simulink model "Inverter_Trifase_PWM_23"  (R2023b)
settings: Solver=ode23s  StartTime=0.0  StopTime=5
values from neighbouring files (symbols this model uses):
  Lc = 10e-3    (= 0.01)    [data.m]
  Rc = 20    [data.m]
  tau = 0.1    [data.m]
  Tc = 100e-6    (= 0.0001)    [data.m]
undefined symbols (not defined in the file or in its folder): DiscIntNeverNeededParam
libraries: fl_lib x80, nesl_utility x51, slpidlib x3, simulink x1
(part 2 of 2)

== system Inverter_Trifase_PWM_23/load ==
  Capacitor : fl_lib/Electrical/Electrical Elements/Capacitor  c=Cc F  r=1e-6 Ohm  g=0 1/Ohm  i_specify=off  i_priority=None  i=0 A  i_nominal_specify=off  i_nominal_value=1  i_nominal_unit=A  v_specify=off  v_priority=None  v=0 V  v_nominal_specify=off  v_nominal_value=1  v_nominal_unit=V  vc_specify=off  vc_priority=High  vc=0 V  vc_nominal_specify=off  vc_nominal_value=1  vc_nominal_unit=V
  Capacitor1 : fl_lib/Electrical/Electrical Elements/Capacitor  c=Cc F  r=1e-6 Ohm  g=0 1/Ohm  i_specify=off  i_priority=None  i=0 A  i_nominal_specify=off  i_nominal_value=1  i_nominal_unit=A  v_specify=off  v_priority=None  v=0 V  v_nominal_specify=off  v_nominal_value=1  v_nominal_unit=V  vc_specify=off  vc_priority=High  vc=0 V  vc_nominal_specify=off  vc_nominal_value=1  vc_nominal_unit=V
  Capacitor2 : fl_lib/Electrical/Electrical Elements/Capacitor  c=Cc F  r=1e-6 Ohm  g=0 1/Ohm  i_specify=off  i_priority=None  i=0 A  i_nominal_specify=off  i_nominal_value=1  i_nominal_unit=A  v_specify=off  v_priority=None  v=0 V  v_nominal_specify=off  v_nominal_value=1  v_nominal_unit=V  vc_specify=off  vc_priority=High  vc=0 V  vc_nominal_specify=off  vc_nominal_value=1  vc_nominal_unit=V
  Electrical Reference1 : fl_lib/Electrical/Electrical Elements/Electrical Reference
  Inductor : fl_lib/Electrical/Electrical Elements/Inductor  l=Lc H  r=0 Ohm  g=1e-9 1/Ohm  i_specify=off  i_priority=None  i=0 A  i_nominal_specify=off  i_nominal_value=1  i_nominal_unit=A  v_specify=off  v_priority=None  v=0 V  v_nominal_specify=off  v_nominal_value=1  v_nominal_unit=V  i_L_specify=on  i_L_priority=High  i_L=0 A  i_L_nominal_specify=off  i_L_nominal_value=1  i_L_nominal_unit=A
  Inductor1 : fl_lib/Electrical/Electrical Elements/Inductor  l=Lc H  r=0 Ohm  g=1e-9 1/Ohm  i_specify=off  i_priority=None  i=0 A  i_nominal_specify=off  i_nominal_value=1  i_nominal_unit=A  v_specify=off  v_priority=None  v=0 V  v_nominal_specify=off  v_nominal_value=1  v_nominal_unit=V  i_L_specify=on  i_L_priority=High  i_L=0 A  i_L_nominal_specify=off  i_L_nominal_value=1  i_L_nominal_unit=A
  Inductor2 : fl_lib/Electrical/Electrical Elements/Inductor  l=Lc H  r=0 Ohm  g=1e-9 1/Ohm  i_specify=off  i_priority=None  i=0 A  i_nominal_specify=off  i_nominal_value=1  i_nominal_unit=A  v_specify=off  v_priority=None  v=0 V  v_nominal_specify=off  v_nominal_value=1  v_nominal_unit=V  i_L_specify=on  i_L_priority=High  i_L=0 A  i_L_nominal_specify=off  i_L_nominal_value=1  i_L_nominal_unit=A
  Resistor : fl_lib/Electrical/Electrical Elements/Resistor  R=Rc Ohm  i_specify=off  i_priority=None  i=0 A  i_nominal_specify=off  i_nominal_value=1  i_nominal_unit=A  v_specify=off  v_priority=None  v=0 V  v_nominal_specify=off  v_nominal_value=1  v_nominal_unit=V
  Resistor1 : fl_lib/Electrical/Electrical Elements/Resistor  R=Rc Ohm  i_specify=off  i_priority=None  i=0 A  i_nominal_specify=off  i_nominal_value=1  i_nominal_unit=A  v_specify=off  v_priority=None  v=0 V  v_nominal_specify=off  v_nominal_value=1  v_nominal_unit=V
  Resistor2 : fl_lib/Electrical/Electrical Elements/Resistor  R=Rc Ohm  i_specify=off  i_priority=None  i=0 A  i_nominal_specify=off  i_nominal_value=1  i_nominal_unit=A  v_specify=off  v_priority=None  v=0 V  v_nominal_specify=off  v_nominal_value=1  v_nominal_unit=V
  A : PMIOPort  Side=Left
  B : PMIOPort  Port=2  Side=Left
  C : PMIOPort  Port=3  Side=Left
  connections:
  Inductor/RConn1 -- Electrical Reference1/LConn1 -- Inductor2/RConn1 -- Inductor1/RConn1
  Inductor/LConn1 -- Resistor/RConn1
  Inductor1/LConn1 -- Resistor1/RConn1
  Inductor2/LConn1 -- Resistor2/RConn1
  Capacitor/LConn1 -- A/RConn1
  Capacitor/RConn1 -- Resistor/LConn1
  Capacitor1/LConn1 -- B/RConn1
  Capacitor1/RConn1 -- Resistor1/LConn1
  Capacitor2/LConn1 -- C/RConn1
  Capacitor2/RConn1 -- Resistor2/LConn1

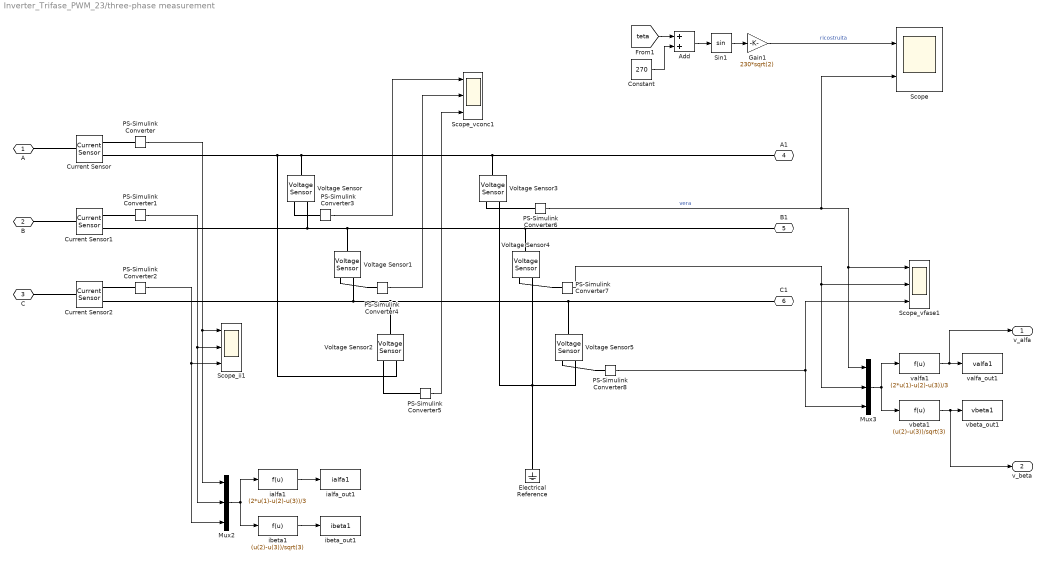
== system Inverter_Trifase_PWM_23/three-phase measurement ==
  Add : Sum
  Constant : Constant  Value=270
  Current Sensor : fl_lib/Electrical/Electrical Sensors/Current Sensor
  Current Sensor1 : fl_lib/Electrical/Electrical Sensors/Current Sensor
  Current Sensor2 : fl_lib/Electrical/Electrical Sensors/Current Sensor
  Electrical Reference : fl_lib/Electrical/Electrical Elements/Electrical Reference
  Gain1 : Gain  Gain=230*sqrt(2)
  Mux2 : Mux  Inputs=3
  Mux3 : Mux  Inputs=3
  PS-Simulink Converter{,1..8} (9 alike) : nesl_utility/PS-Simulink Converter  PhysicalDomain=network_engine_domain  SubClassName=ps_output  LeftPortType=input  RightPortType=output  PseudoPeriodic=off  Frequencies=[]  VectorFormat=inherit  Unit=inherit  AffineConversion=off
  Scope : Scope  NumInputPorts=2
  Scope_ii1 : Scope  NumInputPorts=3
  Scope_vconc1 : Scope  NumInputPorts=3
  Scope_vfase1 : Scope  NumInputPorts=3
  Sin1 : Trigonometry
  Voltage Sensor{,1..5} (6 alike) : fl_lib/Electrical/Electrical Sensors/Voltage Sensor
  ialfa1 : Fcn  Expr=(2*u(1)-u(2)-u(3))/3
  ialfa_out1 : ToWorkspace  VariableName=ialfa1  SampleTime=-1
  ibeta1 : Fcn  Expr=(u(2)-u(3))/sqrt(3)
  ibeta_out1 : ToWorkspace  VariableName=ibeta1  SampleTime=-1
  valfa1 : Fcn  Expr=(2*u(1)-u(2)-u(3))/3
  valfa_out1 : ToWorkspace  VariableName=valfa1  SampleTime=-1
  vbeta1 : Fcn  Expr=(u(2)-u(3))/sqrt(3)
  vbeta_out1 : ToWorkspace  VariableName=vbeta1  SampleTime=-1
  A : PMIOPort  Side=Left
  B : PMIOPort  Port=2  Side=Left
  C : PMIOPort  Port=3  Side=Left
  A1 : PMIOPort  Port=4  Side=Right
  B1 : PMIOPort  Port=5  Side=Right
  C1 : PMIOPort  Port=6  Side=Right
  v_alfa : Outport
  v_beta : Outport  Port=2
  wires:
  ibeta1/1 -> ibeta_out1/1
  ialfa1/1 -> ialfa_out1/1
  Mux2/1 -> ialfa1/1, ibeta1/1
  PS-Simulink Converter2/1 -> Scope_ii1/3, Mux2/3
  PS-Simulink Converter1/1 -> Scope_ii1/2, Mux2/2
  PS-Simulink Converter/1 -> Scope_ii1/1, Mux2/1
  PS-Simulink Converter3/1 -> Scope_vconc1/1
  PS-Simulink Converter4/1 -> Scope_vconc1/2
  PS-Simulink Converter5/1 -> Scope_vconc1/3
  vbeta1/1 -> v_beta/1, vbeta_out1/1
  valfa1/1 -> v_alfa/1, valfa_out1/1
  Mux3/1 -> valfa1/1, vbeta1/1
  PS-Simulink Converter6/1 -> Scope/2, Scope_vfase1/1, Mux3/1  "vera"
  PS-Simulink Converter7/1 -> Scope_vfase1/2, Mux3/2
  PS-Simulink Converter8/1 -> Mux3/3, Scope_vfase1/3
  Gain1/1 -> Scope/1  "ricostruita"
  Sin1/1 -> Gain1/1
  Constant/1 -> Add/2
  [teta] -> Add/1
  Add/1 -> Sin1/1
  connections:
  Current Sensor/LConn1 -- A/RConn1
  Current Sensor1/LConn1 -- B/RConn1
  C/RConn1 -- Current Sensor2/LConn1
  PS-Simulink Converter/LConn1 -- Current Sensor/RConn1
  PS-Simulink Converter1/LConn1 -- Current Sensor1/RConn1
  PS-Simulink Converter2/LConn1 -- Current Sensor2/RConn1
  A1/RConn1 -- Voltage Sensor3/LConn1 -- Voltage Sensor/LConn1 -- Voltage Sensor2/RConn2 -- Current Sensor/RConn2
  B1/RConn1 -- Voltage Sensor1/LConn1 -- Voltage Sensor/RConn2 -- Current Sensor1/RConn2 -- Voltage Sensor4/LConn1
  C1/RConn1 -- Voltage Sensor5/LConn1 -- Voltage Sensor2/LConn1 -- Voltage Sensor1/RConn2 -- Current Sensor2/RConn2
  PS-Simulink Converter3/LConn1 -- Voltage Sensor/RConn1
  PS-Simulink Converter4/LConn1 -- Voltage Sensor1/RConn1
  PS-Simulink Converter5/LConn1 -- Voltage Sensor2/RConn1
  Voltage Sensor3/RConn2 -- Electrical Reference/LConn1 -- Voltage Sensor5/RConn2 -- Voltage Sensor4/RConn2
  PS-Simulink Converter6/LConn1 -- Voltage Sensor3/RConn1
  PS-Simulink Converter7/LConn1 -- Voltage Sensor4/RConn1
  PS-Simulink Converter8/LConn1 -- Voltage Sensor5/RConn1

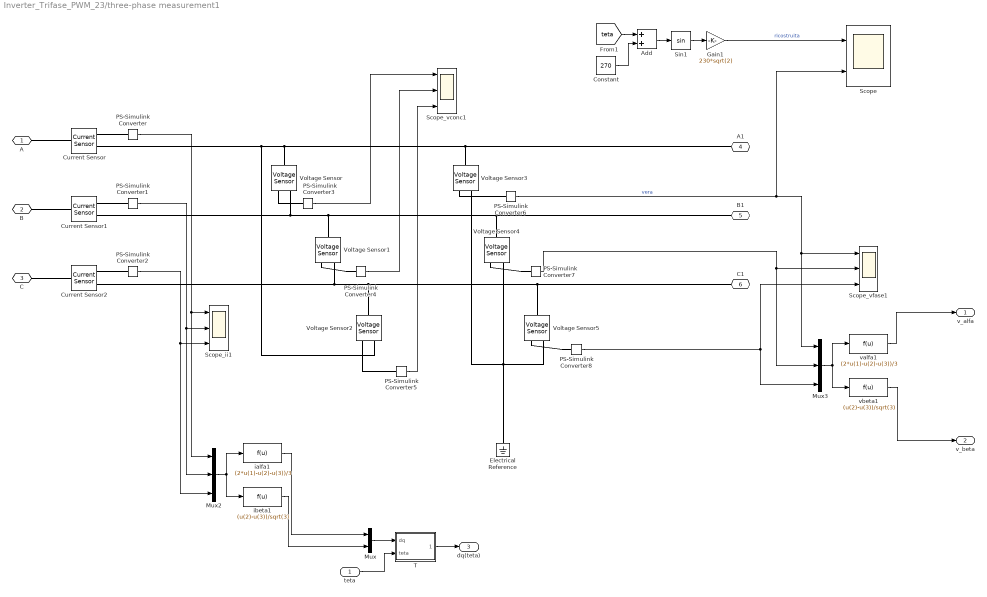
== system Inverter_Trifase_PWM_23/three-phase measurement1 ==
  teta : Inport
  Add : Sum
  Constant : Constant  Value=270
  Current Sensor : fl_lib/Electrical/Electrical Sensors/Current Sensor
  Current Sensor1 : fl_lib/Electrical/Electrical Sensors/Current Sensor
  Current Sensor2 : fl_lib/Electrical/Electrical Sensors/Current Sensor
  Electrical Reference : fl_lib/Electrical/Electrical Elements/Electrical Reference
  Gain1 : Gain  Gain=230*sqrt(2)
  Mux : Mux  Inputs=2
  Mux2 : Mux  Inputs=3
  Mux3 : Mux  Inputs=3
  PS-Simulink Converter{,1..8} (9 alike) : nesl_utility/PS-Simulink Converter  PhysicalDomain=network_engine_domain  SubClassName=ps_output  LeftPortType=input  RightPortType=output  PseudoPeriodic=off  Frequencies=[]  VectorFormat=inherit  Unit=inherit  AffineConversion=off
  Scope : Scope  NumInputPorts=2
  Scope_ii1 : Scope  NumInputPorts=3
  Scope_vconc1 : Scope  NumInputPorts=3
  Scope_vfase1 : Scope  NumInputPorts=3
  Sin1 : Trigonometry
  T : Subsystem
  Voltage Sensor{,1..5} (6 alike) : fl_lib/Electrical/Electrical Sensors/Voltage Sensor
  ialfa1 : Fcn  Expr=(2*u(1)-u(2)-u(3))/3
  ibeta1 : Fcn  Expr=(u(2)-u(3))/sqrt(3)
  valfa1 : Fcn  Expr=(2*u(1)-u(2)-u(3))/3
  vbeta1 : Fcn  Expr=(u(2)-u(3))/sqrt(3)
  A : PMIOPort  Side=Left
  B : PMIOPort  Port=2  Side=Left
  C : PMIOPort  Port=3  Side=Left
  A1 : PMIOPort  Port=4  Side=Right
  B1 : PMIOPort  Port=5  Side=Right
  C1 : PMIOPort  Port=6  Side=Right
  v_alfa : Outport
  v_beta : Outport  Port=2
  dq(teta) : Outport  Port=3
  wires:
  ibeta1/1 -> Mux/2
  ialfa1/1 -> Mux/1
  Mux2/1 -> ialfa1/1, ibeta1/1
  PS-Simulink Converter2/1 -> Scope_ii1/3, Mux2/3
  PS-Simulink Converter1/1 -> Scope_ii1/2, Mux2/2
  PS-Simulink Converter/1 -> Scope_ii1/1, Mux2/1
  PS-Simulink Converter3/1 -> Scope_vconc1/1
  PS-Simulink Converter4/1 -> Scope_vconc1/2
  PS-Simulink Converter5/1 -> Scope_vconc1/3
  vbeta1/1 -> v_beta/1
  valfa1/1 -> v_alfa/1
  Mux3/1 -> valfa1/1, vbeta1/1
  PS-Simulink Converter6/1 -> Scope/2, Scope_vfase1/1, Mux3/1  "vera"
  PS-Simulink Converter7/1 -> Scope_vfase1/2, Mux3/2
  PS-Simulink Converter8/1 -> Mux3/3, Scope_vfase1/3
  Gain1/1 -> Scope/1  "ricostruita"
  Sin1/1 -> Gain1/1
  Constant/1 -> Add/2
  [teta] -> Add/1
  Add/1 -> Sin1/1
  Mux/1 -> T/1(dq)
  teta/1 -> T/2(teta)
  T/1(dq(teta)) -> dq(teta)/1
  connections:
  Current Sensor/LConn1 -- A/RConn1
  Current Sensor1/LConn1 -- B/RConn1
  C/RConn1 -- Current Sensor2/LConn1
  PS-Simulink Converter/LConn1 -- Current Sensor/RConn1
  PS-Simulink Converter1/LConn1 -- Current Sensor1/RConn1
  PS-Simulink Converter2/LConn1 -- Current Sensor2/RConn1
  A1/RConn1 -- Voltage Sensor3/LConn1 -- Voltage Sensor/LConn1 -- Voltage Sensor2/RConn2 -- Current Sensor/RConn2
  B1/RConn1 -- Voltage Sensor1/LConn1 -- Voltage Sensor/RConn2 -- Current Sensor1/RConn2 -- Voltage Sensor4/LConn1
  C1/RConn1 -- Voltage Sensor5/LConn1 -- Voltage Sensor2/LConn1 -- Voltage Sensor1/RConn2 -- Current Sensor2/RConn2
  PS-Simulink Converter3/LConn1 -- Voltage Sensor/RConn1
  PS-Simulink Converter4/LConn1 -- Voltage Sensor1/RConn1
  PS-Simulink Converter5/LConn1 -- Voltage Sensor2/RConn1
  Voltage Sensor3/RConn2 -- Electrical Reference/LConn1 -- Voltage Sensor5/RConn2 -- Voltage Sensor4/RConn2
  PS-Simulink Converter6/LConn1 -- Voltage Sensor3/RConn1
  PS-Simulink Converter7/LConn1 -- Voltage Sensor4/RConn1
  PS-Simulink Converter8/LConn1 -- Voltage Sensor5/RConn1

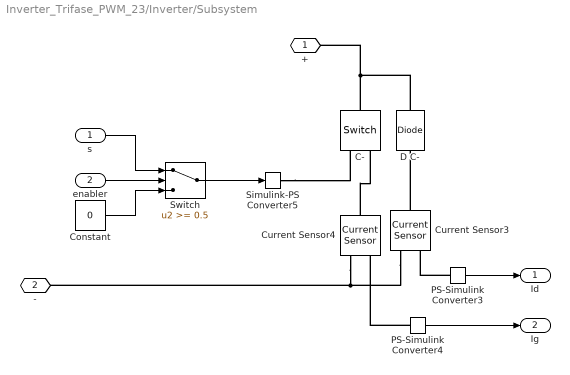
== system Inverter_Trifase_PWM_23/Inverter/Subsystem ==
  s : Inport
  enabler : Inport  Port=2
  C- : fl_lib/Electrical/Electrical Elements/Switch  R_closed=0.01 Ohm  G_open=1e-8 1/Ohm  Threshold=0.5  i_specify=off  i_priority=None  i=0 A  i_nominal_specify=off  i_nominal_value=1  i_nominal_unit=A  v_specify=off  v_priority=None  v=0 V  v_nominal_specify=off  v_nominal_value=1  v_nominal_unit=V
  Constant : Constant  Value=0
  Current Sensor3 : fl_lib/Electrical/Electrical Sensors/Current Sensor
  Current Sensor4 : fl_lib/Electrical/Electrical Sensors/Current Sensor
  D C- : fl_lib/Electrical/Electrical Elements/Diode  Vf=0.6 V  Ron=0.3 Ohm  Goff=1e-8 1/Ohm  i_specify=off  i_priority=None  i=0 A  i_nominal_specify=off  i_nominal_value=1  i_nominal_unit=A  v_specify=off  v_priority=None  v=0 V  v_nominal_specify=off  v_nominal_value=1  v_nominal_unit=V
  PS-Simulink Converter3 : nesl_utility/PS-Simulink Converter  PhysicalDomain=network_engine_domain  SubClassName=ps_output  LeftPortType=input  RightPortType=output  PseudoPeriodic=off  Frequencies=[]  VectorFormat=inherit  Unit=inherit  AffineConversion=off
  PS-Simulink Converter4 : nesl_utility/PS-Simulink Converter  PhysicalDomain=network_engine_domain  SubClassName=ps_output  LeftPortType=input  RightPortType=output  PseudoPeriodic=off  Frequencies=[]  VectorFormat=inherit  Unit=inherit  AffineConversion=off
  Simulink-PS Converter5 : nesl_utility/Simulink-PS Converter  PhysicalDomain=network_engine_domain  SubClassName=ps_input  LeftPortType=input  RightPortType=output  PseudoPeriodic=off  Frequencies=[]  NoiseDistribution=none  NoiseParameters=[]  Unit=1  AffineConversion=off  FilteringAndDerivatives=provide  SimscapeFilterOrder=1  InputFilterTimeConstant=0.001  UdotUserProvided=0
  Switch : Switch  Threshold=0.5  SaturateOnIntegerOverflow=off  InputSameDT=off
  + : PMIOPort  Side=Left
  - : PMIOPort  Port=2  Side=Right
  Id : Outport
  Ig : Outport  Port=2
  wires:
  PS-Simulink Converter3/1 -> Id/1
  PS-Simulink Converter4/1 -> Ig/1
  s/1 -> Switch/1
  Constant/1 -> Switch/3
  enabler/1 -> Switch/2
  Switch/1 -> Simulink-PS Converter5/1
  connections:
  Current Sensor4/LConn1 -- C-/RConn2
  C-/LConn1 -- +/RConn1 -- D C-/RConn1
  PS-Simulink Converter4/LConn1 -- Current Sensor4/RConn1
  Current Sensor3/LConn1 -- D C-/LConn1
  PS-Simulink Converter3/LConn1 -- Current Sensor3/RConn1
  Current Sensor3/RConn2 -- Current Sensor4/RConn2 -- -/RConn1
  Simulink-PS Converter5/RConn1 -- C-/RConn1

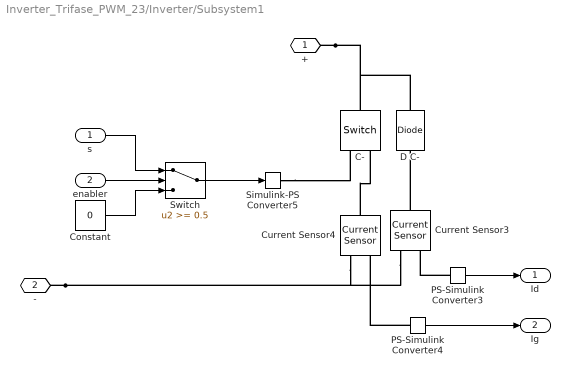
== system Inverter_Trifase_PWM_23/Inverter/Subsystem1 ==
  s : Inport
  enabler : Inport  Port=2
  C- : fl_lib/Electrical/Electrical Elements/Switch  R_closed=0.01 Ohm  G_open=1e-8 1/Ohm  Threshold=0.5  i_specify=off  i_priority=None  i=0 A  i_nominal_specify=off  i_nominal_value=1  i_nominal_unit=A  v_specify=off  v_priority=None  v=0 V  v_nominal_specify=off  v_nominal_value=1  v_nominal_unit=V
  Constant : Constant  Value=0
  Current Sensor3 : fl_lib/Electrical/Electrical Sensors/Current Sensor
  Current Sensor4 : fl_lib/Electrical/Electrical Sensors/Current Sensor
  D C- : fl_lib/Electrical/Electrical Elements/Diode  Vf=0.6 V  Ron=0.3 Ohm  Goff=1e-8 1/Ohm  i_specify=off  i_priority=None  i=0 A  i_nominal_specify=off  i_nominal_value=1  i_nominal_unit=A  v_specify=off  v_priority=None  v=0 V  v_nominal_specify=off  v_nominal_value=1  v_nominal_unit=V
  PS-Simulink Converter3 : nesl_utility/PS-Simulink Converter  PhysicalDomain=network_engine_domain  SubClassName=ps_output  LeftPortType=input  RightPortType=output  PseudoPeriodic=off  Frequencies=[]  VectorFormat=inherit  Unit=inherit  AffineConversion=off
  PS-Simulink Converter4 : nesl_utility/PS-Simulink Converter  PhysicalDomain=network_engine_domain  SubClassName=ps_output  LeftPortType=input  RightPortType=output  PseudoPeriodic=off  Frequencies=[]  VectorFormat=inherit  Unit=inherit  AffineConversion=off
  Simulink-PS Converter5 : nesl_utility/Simulink-PS Converter  PhysicalDomain=network_engine_domain  SubClassName=ps_input  LeftPortType=input  RightPortType=output  PseudoPeriodic=off  Frequencies=[]  NoiseDistribution=none  NoiseParameters=[]  Unit=1  AffineConversion=off  FilteringAndDerivatives=provide  SimscapeFilterOrder=1  InputFilterTimeConstant=0.001  UdotUserProvided=0
  Switch : Switch  Threshold=0.5  SaturateOnIntegerOverflow=off  InputSameDT=off
  + : PMIOPort  Side=Left
  - : PMIOPort  Port=2  Side=Right
  Id : Outport
  Ig : Outport  Port=2
  wires:
  Switch/1 -> Simulink-PS Converter5/1
  enabler/1 -> Switch/2
  Constant/1 -> Switch/3
  s/1 -> Switch/1
  PS-Simulink Converter4/1 -> Ig/1
  PS-Simulink Converter3/1 -> Id/1
  connections:
  Simulink-PS Converter5/RConn1 -- C-/RConn1
  -/RConn1 -- Current Sensor4/RConn2 -- Current Sensor3/RConn2
  PS-Simulink Converter3/LConn1 -- Current Sensor3/RConn1
  Current Sensor3/LConn1 -- D C-/LConn1
  PS-Simulink Converter4/LConn1 -- Current Sensor4/RConn1
  +/RConn1 -- D C-/RConn1 -- C-/LConn1
  Current Sensor4/LConn1 -- C-/RConn2

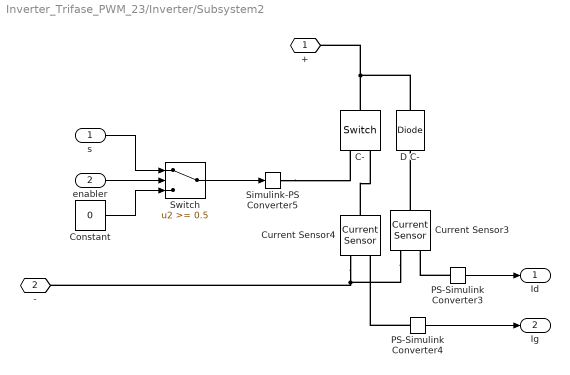
== system Inverter_Trifase_PWM_23/Inverter/Subsystem2 ==
  s : Inport
  enabler : Inport  Port=2
  C- : fl_lib/Electrical/Electrical Elements/Switch  R_closed=0.01 Ohm  G_open=1e-8 1/Ohm  Threshold=0.5  i_specify=off  i_priority=None  i=0 A  i_nominal_specify=off  i_nominal_value=1  i_nominal_unit=A  v_specify=off  v_priority=None  v=0 V  v_nominal_specify=off  v_nominal_value=1  v_nominal_unit=V
  Constant : Constant  Value=0
  Current Sensor3 : fl_lib/Electrical/Electrical Sensors/Current Sensor
  Current Sensor4 : fl_lib/Electrical/Electrical Sensors/Current Sensor
  D C- : fl_lib/Electrical/Electrical Elements/Diode  Vf=0.6 V  Ron=0.3 Ohm  Goff=1e-8 1/Ohm  i_specify=off  i_priority=None  i=0 A  i_nominal_specify=off  i_nominal_value=1  i_nominal_unit=A  v_specify=off  v_priority=None  v=0 V  v_nominal_specify=off  v_nominal_value=1  v_nominal_unit=V
  PS-Simulink Converter3 : nesl_utility/PS-Simulink Converter  PhysicalDomain=network_engine_domain  SubClassName=ps_output  LeftPortType=input  RightPortType=output  PseudoPeriodic=off  Frequencies=[]  VectorFormat=inherit  Unit=inherit  AffineConversion=off
  PS-Simulink Converter4 : nesl_utility/PS-Simulink Converter  PhysicalDomain=network_engine_domain  SubClassName=ps_output  LeftPortType=input  RightPortType=output  PseudoPeriodic=off  Frequencies=[]  VectorFormat=inherit  Unit=inherit  AffineConversion=off
  Simulink-PS Converter5 : nesl_utility/Simulink-PS Converter  PhysicalDomain=network_engine_domain  SubClassName=ps_input  LeftPortType=input  RightPortType=output  PseudoPeriodic=off  Frequencies=[]  NoiseDistribution=none  NoiseParameters=[]  Unit=1  AffineConversion=off  FilteringAndDerivatives=provide  SimscapeFilterOrder=1  InputFilterTimeConstant=0.001  UdotUserProvided=0
  Switch : Switch  Threshold=0.5  SaturateOnIntegerOverflow=off  InputSameDT=off
  + : PMIOPort  Side=Left
  - : PMIOPort  Port=2  Side=Right
  Id : Outport
  Ig : Outport  Port=2
  wires:
  PS-Simulink Converter3/1 -> Id/1
  PS-Simulink Converter4/1 -> Ig/1
  s/1 -> Switch/1
  Constant/1 -> Switch/3
  enabler/1 -> Switch/2
  Switch/1 -> Simulink-PS Converter5/1
  connections:
  Current Sensor4/LConn1 -- C-/RConn2
  C-/LConn1 -- D C-/RConn1 -- +/RConn1
  PS-Simulink Converter4/LConn1 -- Current Sensor4/RConn1
  Current Sensor3/LConn1 -- D C-/LConn1
  PS-Simulink Converter3/LConn1 -- Current Sensor3/RConn1
  Current Sensor3/RConn2 -- Current Sensor4/RConn2 -- -/RConn1
  Simulink-PS Converter5/RConn1 -- C-/RConn1

== system Inverter_Trifase_PWM_23/Inverter/Subsystem3 ==
  s : Inport
  enabler : Inport  Port=2
  C- : fl_lib/Electrical/Electrical Elements/Switch  R_closed=0.01 Ohm  G_open=1e-8 1/Ohm  Threshold=0.5  i_specify=off  i_priority=None  i=0 A  i_nominal_specify=off  i_nominal_value=1  i_nominal_unit=A  v_specify=off  v_priority=None  v=0 V  v_nominal_specify=off  v_nominal_value=1  v_nominal_unit=V
  Constant : Constant  Value=0
  Current Sensor3 : fl_lib/Electrical/Electrical Sensors/Current Sensor
  Current Sensor4 : fl_lib/Electrical/Electrical Sensors/Current Sensor
  D C- : fl_lib/Electrical/Electrical Elements/Diode  Vf=0.6 V  Ron=0.3 Ohm  Goff=1e-8 1/Ohm  i_specify=off  i_priority=None  i=0 A  i_nominal_specify=off  i_nominal_value=1  i_nominal_unit=A  v_specify=off  v_priority=None  v=0 V  v_nominal_specify=off  v_nominal_value=1  v_nominal_unit=V
  PS-Simulink Converter3 : nesl_utility/PS-Simulink Converter  PhysicalDomain=network_engine_domain  SubClassName=ps_output  LeftPortType=input  RightPortType=output  PseudoPeriodic=off  Frequencies=[]  VectorFormat=inherit  Unit=inherit  AffineConversion=off
  PS-Simulink Converter4 : nesl_utility/PS-Simulink Converter  PhysicalDomain=network_engine_domain  SubClassName=ps_output  LeftPortType=input  RightPortType=output  PseudoPeriodic=off  Frequencies=[]  VectorFormat=inherit  Unit=inherit  AffineConversion=off
  Simulink-PS Converter5 : nesl_utility/Simulink-PS Converter  PhysicalDomain=network_engine_domain  SubClassName=ps_input  LeftPortType=input  RightPortType=output  PseudoPeriodic=off  Frequencies=[]  NoiseDistribution=none  NoiseParameters=[]  Unit=1  AffineConversion=off  FilteringAndDerivatives=provide  SimscapeFilterOrder=1  InputFilterTimeConstant=0.001  UdotUserProvided=0
  Switch : Switch  Threshold=0.5  SaturateOnIntegerOverflow=off  InputSameDT=off
  + : PMIOPort  Side=Left
  - : PMIOPort  Port=2  Side=Right
  Id : Outport
  Ig : Outport  Port=2
  wires:
  Switch/1 -> Simulink-PS Converter5/1
  enabler/1 -> Switch/2
  Constant/1 -> Switch/3
  s/1 -> Switch/1
  PS-Simulink Converter4/1 -> Ig/1
  PS-Simulink Converter3/1 -> Id/1
  connections:
  Simulink-PS Converter5/RConn1 -- C-/RConn1
  -/RConn1 -- Current Sensor4/RConn2 -- Current Sensor3/RConn2
  PS-Simulink Converter3/LConn1 -- Current Sensor3/RConn1
  Current Sensor3/LConn1 -- D C-/LConn1
  PS-Simulink Converter4/LConn1 -- Current Sensor4/RConn1
  +/RConn1 -- D C-/RConn1 -- C-/LConn1
  Current Sensor4/LConn1 -- C-/RConn2

== system Inverter_Trifase_PWM_23/Inverter/Subsystem4 ==
  s : Inport
  enabler : Inport  Port=2
  C- : fl_lib/Electrical/Electrical Elements/Switch  R_closed=0.01 Ohm  G_open=1e-8 1/Ohm  Threshold=0.5  i_specify=off  i_priority=None  i=0 A  i_nominal_specify=off  i_nominal_value=1  i_nominal_unit=A  v_specify=off  v_priority=None  v=0 V  v_nominal_specify=off  v_nominal_value=1  v_nominal_unit=V
  Constant : Constant  Value=0
  Current Sensor3 : fl_lib/Electrical/Electrical Sensors/Current Sensor
  Current Sensor4 : fl_lib/Electrical/Electrical Sensors/Current Sensor
  D C- : fl_lib/Electrical/Electrical Elements/Diode  Vf=0.6 V  Ron=0.3 Ohm  Goff=1e-8 1/Ohm  i_specify=off  i_priority=None  i=0 A  i_nominal_specify=off  i_nominal_value=1  i_nominal_unit=A  v_specify=off  v_priority=None  v=0 V  v_nominal_specify=off  v_nominal_value=1  v_nominal_unit=V
  PS-Simulink Converter3 : nesl_utility/PS-Simulink Converter  PhysicalDomain=network_engine_domain  SubClassName=ps_output  LeftPortType=input  RightPortType=output  PseudoPeriodic=off  Frequencies=[]  VectorFormat=inherit  Unit=inherit  AffineConversion=off
  PS-Simulink Converter4 : nesl_utility/PS-Simulink Converter  PhysicalDomain=network_engine_domain  SubClassName=ps_output  LeftPortType=input  RightPortType=output  PseudoPeriodic=off  Frequencies=[]  VectorFormat=inherit  Unit=inherit  AffineConversion=off
  Simulink-PS Converter5 : nesl_utility/Simulink-PS Converter  PhysicalDomain=network_engine_domain  SubClassName=ps_input  LeftPortType=input  RightPortType=output  PseudoPeriodic=off  Frequencies=[]  NoiseDistribution=none  NoiseParameters=[]  Unit=1  AffineConversion=off  FilteringAndDerivatives=provide  SimscapeFilterOrder=1  InputFilterTimeConstant=0.001  UdotUserProvided=0
  Switch : Switch  Threshold=0.5  SaturateOnIntegerOverflow=off  InputSameDT=off
  + : PMIOPort  Side=Left
  - : PMIOPort  Port=2  Side=Right
  Id : Outport
  Ig : Outport  Port=2
  wires:
  Switch/1 -> Simulink-PS Converter5/1
  enabler/1 -> Switch/2
  Constant/1 -> Switch/3
  s/1 -> Switch/1
  PS-Simulink Converter4/1 -> Ig/1
  PS-Simulink Converter3/1 -> Id/1
  connections:
  Simulink-PS Converter5/RConn1 -- C-/RConn1
  -/RConn1 -- Current Sensor4/RConn2 -- Current Sensor3/RConn2
  PS-Simulink Converter3/LConn1 -- Current Sensor3/RConn1
  Current Sensor3/LConn1 -- D C-/LConn1
  PS-Simulink Converter4/LConn1 -- Current Sensor4/RConn1
  +/RConn1 -- D C-/RConn1 -- C-/LConn1
  Current Sensor4/LConn1 -- C-/RConn2

== system Inverter_Trifase_PWM_23/Inverter/Subsystem5 ==
  s : Inport
  enabler : Inport  Port=2
  C- : fl_lib/Electrical/Electrical Elements/Switch  R_closed=0.01 Ohm  G_open=1e-8 1/Ohm  Threshold=0.5  i_specify=off  i_priority=None  i=0 A  i_nominal_specify=off  i_nominal_value=1  i_nominal_unit=A  v_specify=off  v_priority=None  v=0 V  v_nominal_specify=off  v_nominal_value=1  v_nominal_unit=V
  Constant : Constant  Value=0
  Current Sensor3 : fl_lib/Electrical/Electrical Sensors/Current Sensor
  Current Sensor4 : fl_lib/Electrical/Electrical Sensors/Current Sensor
  D C- : fl_lib/Electrical/Electrical Elements/Diode  Vf=0.6 V  Ron=0.3 Ohm  Goff=1e-8 1/Ohm  i_specify=off  i_priority=None  i=0 A  i_nominal_specify=off  i_nominal_value=1  i_nominal_unit=A  v_specify=off  v_priority=None  v=0 V  v_nominal_specify=off  v_nominal_value=1  v_nominal_unit=V
  PS-Simulink Converter3 : nesl_utility/PS-Simulink Converter  PhysicalDomain=network_engine_domain  SubClassName=ps_output  LeftPortType=input  RightPortType=output  PseudoPeriodic=off  Frequencies=[]  VectorFormat=inherit  Unit=inherit  AffineConversion=off
  PS-Simulink Converter4 : nesl_utility/PS-Simulink Converter  PhysicalDomain=network_engine_domain  SubClassName=ps_output  LeftPortType=input  RightPortType=output  PseudoPeriodic=off  Frequencies=[]  VectorFormat=inherit  Unit=inherit  AffineConversion=off
  Simulink-PS Converter5 : nesl_utility/Simulink-PS Converter  PhysicalDomain=network_engine_domain  SubClassName=ps_input  LeftPortType=input  RightPortType=output  PseudoPeriodic=off  Frequencies=[]  NoiseDistribution=none  NoiseParameters=[]  Unit=1  AffineConversion=off  FilteringAndDerivatives=provide  SimscapeFilterOrder=1  InputFilterTimeConstant=0.001  UdotUserProvided=0
  Switch : Switch  Threshold=0.5  SaturateOnIntegerOverflow=off  InputSameDT=off
  + : PMIOPort  Side=Left
  - : PMIOPort  Port=2  Side=Right
  Id : Outport
  Ig : Outport  Port=2
  wires:
  PS-Simulink Converter3/1 -> Id/1
  PS-Simulink Converter4/1 -> Ig/1
  s/1 -> Switch/1
  Constant/1 -> Switch/3
  enabler/1 -> Switch/2
  Switch/1 -> Simulink-PS Converter5/1
  connections:
  Current Sensor4/LConn1 -- C-/RConn2
  C-/LConn1 -- D C-/RConn1 -- +/RConn1
  PS-Simulink Converter4/LConn1 -- Current Sensor4/RConn1
  Current Sensor3/LConn1 -- D C-/LConn1
  PS-Simulink Converter3/LConn1 -- Current Sensor3/RConn1
  Current Sensor3/RConn2 -- Current Sensor4/RConn2 -- -/RConn1
  Simulink-PS Converter5/RConn1 -- C-/RConn1

== system Inverter_Trifase_PWM_23/Modulatore PWM Sinusoidale/A ==
  mA : Inport
  Portante : Inport  Port=2
  Add : Sum  Inputs=+-
  Constant : Constant
  Constant1 : Constant  Value=0
  Switch : Switch  SaturateOnIntegerOverflow=off  InputSameDT=off
  sA : Outport  VectorParamsAs1DForOutWhenUnconnected=off
  wires:
  Constant/1 -> Switch/1
  Constant1/1 -> Switch/3
  mA/1 -> Add/1
  Portante/1 -> Add/2
  Add/1 -> Switch/2
  Switch/1 -> sA/1

== system Inverter_Trifase_PWM_23/Modulatore PWM Sinusoidale/B ==
  mB : Inport
  Portante : Inport  Port=2
  Add : Sum  Inputs=+-
  Constant : Constant
  Constant1 : Constant  Value=0
  Switch : Switch  SaturateOnIntegerOverflow=off  InputSameDT=off
  sB : Outport  VectorParamsAs1DForOutWhenUnconnected=off
  wires:
  Constant/1 -> Switch/1
  Constant1/1 -> Switch/3
  mB/1 -> Add/1
  Portante/1 -> Add/2
  Add/1 -> Switch/2
  Switch/1 -> sB/1

== system Inverter_Trifase_PWM_23/Modulatore PWM Sinusoidale/C ==
  mB : Inport
  Portante : Inport  Port=2
  Add : Sum  Inputs=+-
  Constant : Constant
  Constant1 : Constant  Value=0
  Switch : Switch  SaturateOnIntegerOverflow=off  InputSameDT=off
  sB : Outport  VectorParamsAs1DForOutWhenUnconnected=off
  wires:
  Constant/1 -> Switch/1
  Constant1/1 -> Switch/3
  mB/1 -> Add/1
  Portante/1 -> Add/2
  Add/1 -> Switch/2
  Switch/1 -> sB/1

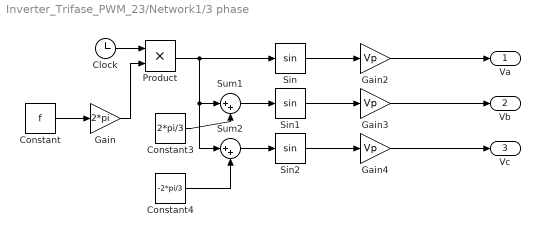
== system Inverter_Trifase_PWM_23/Network1/3 phase ==
  Clock : Clock
  Constant : Constant  Value=f
  Constant3 : Constant  Value=2*pi/3
  Constant4 : Constant  Value=-2*pi/3
  Gain : Gain  Gain=2*pi
  Gain2 : Gain  Gain=Vp
  Gain3 : Gain  Gain=Vp
  Gain4 : Gain  Gain=Vp
  Product : Product
  Sin : Trigonometry
  Sin1 : Trigonometry
  Sin2 : Trigonometry
  Sum1 : Sum  Inputs=|++
  Sum2 : Sum  Inputs=|++
  Va : Outport
  Vb : Outport  Port=2
  Vc : Outport  Port=3
  wires:
  Gain4/1 -> Vc/1
  Gain3/1 -> Vb/1
  Sin1/1 -> Gain3/1
  Constant/1 -> Gain/1
  Gain/1 -> Product/2
  Clock/1 -> Product/1
  Sin/1 -> Gain2/1
  Gain2/1 -> Va/1
  Sum1/1 -> Sin1/1
  Sum2/1 -> Sin2/1
  Sin2/1 -> Gain4/1
  Constant3/1 -> Sum1/2
  Constant4/1 -> Sum2/2
  Product/1 -> Sum1/1, Sum2/1, Sin/1

== system Inverter_Trifase_PWM_23/PLL/D1 ==
  ab(c) : Inport
  Gain : Gain  Gain=[1 0; 1/sqrt(3) 2/sqrt(3)]  Multiplication=Matrix(K*u)
  dq(0) : Outport
  wires:
  Gain/1 -> dq(0)/1
  ab(c)/1 -> Gain/1

== system Inverter_Trifase_PWM_23/PLL/T ==
  dq : Inport
  teta : Inport  Port=2
  Demux : Demux  Outputs=2
  Fcn : Fcn  Expr=cos(u[3])*u[1]+sin(u[3])*u[2]
  Fcn1 : Fcn  Expr=-sin(u[3])*u[1]+cos(u[3])*u[2]
  Mux : Mux  Inputs=3
  Mux1 : Mux  Inputs=2
  dq(teta) : Outport
  wires:
  dq/1 -> Demux/1
  Demux/1 -> Mux/1
  Demux/2 -> Mux/2
  teta/1 -> Mux/3
  Mux/1 -> Fcn1/1, Fcn/1
  Fcn/1 -> Mux1/1
  Fcn1/1 -> Mux1/2
  Mux1/1 -> dq(teta)/1

== system Inverter_Trifase_PWM_23/PLL1/D1 ==
  ab(c) : Inport
  Gain : Gain  Gain=[1 0; 1/sqrt(3) 2/sqrt(3)]  Multiplication=Matrix(K*u)
  dq(0) : Outport
  wires:
  ab(c)/1 -> Gain/1
  Gain/1 -> dq(0)/1

== system Inverter_Trifase_PWM_23/PLL1/Integratore discreto con reset a 2*pi ==
  omega : Inport
  Add : Sum
  Compare To Zero : simulink/Logic and Bit Operations/Compare To Zero  relop=>  OutDataTypeStr=uint8  ZeroCross=off
  Constant : Constant  Value=2*pi
  Constant1 : Constant  Value=-2*pi
  Constant2 : Constant  Value=-2*pi
  Constant3 : Constant  Value=2*pi
  Discrete-Time Integrator : DiscreteIntegrator  ExternalReset=rising  InitialConditionSource=external  SampleTime=-1  ShowStatePort=on  ICPrevOutput=DiscIntNeverNeededParam  ICPrevScaledInput=DiscIntNeverNeededParam
  Logical Operator2 : Logic  Operator=OR  AllPortsSameDT=off  OutDataTypeStr=boolean
  Relational Operator : RelationalOperator  Operator=<=  OutDataTypeStr=boolean  InputSameDT=off
  Relational Operator1 : RelationalOperator  Operator=<=  OutDataTypeStr=boolean  InputSameDT=off
  Switch : Switch  Threshold=0.5  SaturateOnIntegerOverflow=off  InputSameDT=off
  teta : Outport
  wires:
  Logical Operator2/1 -> Discrete-Time Integrator/2
  Relational Operator/1 -> Logical Operator2/1
  Relational Operator1/1 -> Logical Operator2/2
  Discrete-Time Integrator/State -> Add/1, Compare To Zero/1, Relational Operator1/1, Relational Operator/2
  Constant/1 -> Relational Operator/1
  Constant1/1 -> Relational Operator1/2
  omega/1 -> Discrete-Time Integrator/1
  Discrete-Time Integrator/1 -> teta/1
  Constant2/1 -> Switch/1
  Constant3/1 -> Switch/3
  Switch/1 -> Add/2
  Compare To Zero/1 -> Switch/2
  Add/1 -> Discrete-Time Integrator/3

== system Inverter_Trifase_PWM_23/PLL1/PI antiwindup ==
  In : Inport
  Constant : Constant  Value=kp_PLL_edit
  Constant1 : Constant  Value=ki_PLL_edit
  Constant2 : Constant  Value=min_PLL
  Constant3 : Constant  Value=max_PLL
  Embedded MATLAB Function : MATLAB Function  TreatAsAtomicUnit=on
  Out : Outport
  wires:
  Embedded MATLAB Function/1(out) -> Out/1
  Constant3/1 -> Embedded MATLAB Function/5(max)
  Constant2/1 -> Embedded MATLAB Function/4(min)
  Constant1/1 -> Embedded MATLAB Function/3(ki)
  Constant/1 -> Embedded MATLAB Function/2(kp)
  In/1 -> Embedded MATLAB Function/1(error)

== system Inverter_Trifase_PWM_23/PLL1/T ==
  dq : Inport
  teta : Inport  Port=2
  Demux : Demux  Outputs=2
  Fcn : Fcn  Expr=cos(u[3])*u[1]+sin(u[3])*u[2]
  Fcn1 : Fcn  Expr=-sin(u[3])*u[1]+cos(u[3])*u[2]
  Mux : Mux  Inputs=3
  Mux1 : Mux  Inputs=2
  dq(teta) : Outport
  wires:
  Mux1/1 -> dq(teta)/1
  Fcn1/1 -> Mux1/2
  Fcn/1 -> Mux1/1
  Mux/1 -> Fcn/1, Fcn1/1
  teta/1 -> Mux/3
  Demux/2 -> Mux/2
  Demux/1 -> Mux/1
  dq/1 -> Demux/1

== system Inverter_Trifase_PWM_23/three-phase measurement1/T ==
  dq : Inport
  teta : Inport  Port=2
  Demux : Demux  Outputs=2
  Fcn : Fcn  Expr=cos(u[3])*u[1]+sin(u[3])*u[2]
  Fcn1 : Fcn  Expr=-sin(u[3])*u[1]+cos(u[3])*u[2]
  Mux : Mux  Inputs=3
  Mux1 : Mux  Inputs=2
  dq(teta) : Outport
  wires:
  Mux1/1 -> dq(teta)/1
  Fcn1/1 -> Mux1/2
  Fcn/1 -> Mux1/1
  Mux/1 -> Fcn/1, Fcn1/1
  teta/1 -> Mux/3
  Demux/2 -> Mux/2
  Demux/1 -> Mux/1
  dq/1 -> Demux/1

== matlab function Inverter_Trifase_PWM_23/PLL1/PI antiwindup/Embedded MATLAB Function ==
  data: error input; out output; kp input; ki input; min input; max input; Tc parameter
function out = fcn(error,kp,ki,min,max,Tc)
% Regolatore PI con antiwindup.
% Discretizzazione con Eulero all'indietro.

persistent start
persistent error_p
persistent out_p

if (isempty(start))
    start=1;
    error_p=0;
    out_p=0;
end

out=out_p+kp*(error-error_p)+ki*error*Tc;

if out>max
    out=max;
    error=(max-out_p+(kp*error_p))/(kp+(ki*Tc));
elseif out<min
    out=min;
    error=(min-out_p+(kp*error_p))/(kp+(ki*Tc));
end

out_p=out;
error_p=error;
